simulink model "Assignment1_A1V1"  (R2020a)
settings: Solver=FixedStepAuto  StartTime=0.0  StopTime=10.0  FixedStep=1e-3  RelTol=1e-3  EnableMultiTasking=on
undefined symbols (not defined in the file): D10, D11, D12, D2, D4, D5, D7, D8, D9, PTA0, PTA2, PTB23, PTB9, PTC3, PTC4, PTD0, PTD2, PTD3
libraries: frdmk64flib x12
settings Model: ExtModeTrigDuration=5  Creator=Daniyal  LastModifiedBy=Daniyal
settings OptimizationCC: EnhancedBackFolding=on  PassReuseOutputArgsAs=Individual arguments  ZeroExternalMemoryAtStartup=off  ZeroInternalMemoryAtStartup=off  MaxStackSize=64  OptimizeBlockOrder=speed  DifferentSizesBufferReuse=on  OptimizationCustomize=off  EfficientTunableParamExpr=on
settings DebuggingCC: ParameterTunabilityLossMsg=error
settings HardwareCC: ProdBitPerPointer=32  ProdBitPerSizeT=32  ProdBitPerPtrDiffT=32  ProdLargestAtomicInteger=Long  ProdLargestAtomicFloat=Double  ProdWordSize=32  ProdHWDeviceType=ARM Compatible->ARM Cortex
settings SFSimCC: MATLABDynamicMemAlloc=off
settings RTWCC: SystemTargetFile=ert.tlc  HardwareBoard=NXP FRDM-K64F  TemplateMakefile=ert_default_tmf  Toolchain=GNU Tools for ARM Embedded Processors
settings CodeAppCC: ForceParamTrailComments=on  IgnoreCustomStorageClasses=off  OperatorAnnotations=on  SimulinkDataObjDesc=on  SFDataObjDesc=on  InsertBlockDesc=on

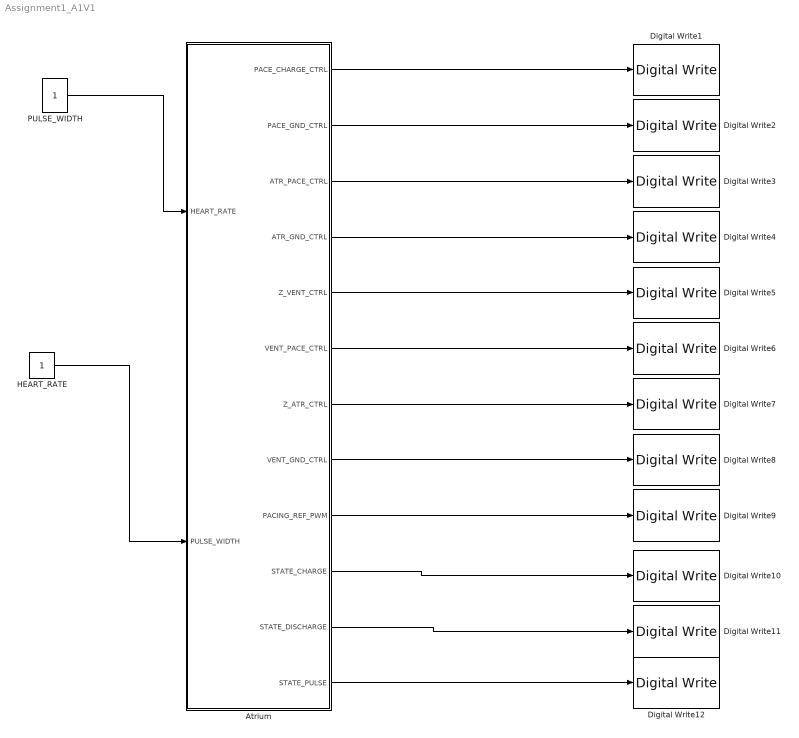
== system Assignment1_A1V1 ==
  Atrium : Stateflow chart  TreatAsAtomicUnit=on
  Digital Write1 : frdmk64flib/Digital Write  Whichpin=PTB9 (D2)
  Digital Write10 : frdmk64flib/Digital Write  Whichpin=RED_LED
  Digital Write11 : frdmk64flib/Digital Write  Whichpin=GREEN_LED
  Digital Write12 : frdmk64flib/Digital Write  Whichpin=BLUE_LED
  Digital Write2 : frdmk64flib/Digital Write  Whichpin=PTD0 (D10)
  Digital Write3 : frdmk64flib/Digital Write  Whichpin=PTA0 (D8)
  Digital Write4 : frdmk64flib/Digital Write  Whichpin=PTD2 (D11)
  Digital Write5 : frdmk64flib/Digital Write  Whichpin=PTC3 (D7)
  Digital Write6 : frdmk64flib/Digital Write  Whichpin=PTC4 (D9)
  Digital Write7 : frdmk64flib/Digital Write  Whichpin=PTB23 (D4)
  Digital Write8 : frdmk64flib/Digital Write  Whichpin=PTD3 (D12)
  Digital Write9 : frdmk64flib/Digital Write  Whichpin=PTA2 (D5)
  HEART_RATE : Constant
  PULSE_WIDTH : Constant
  wires:
  Atrium/4(ATR_GND_CTRL) -> Digital Write4/1
  Atrium/5(Z_VENT_CTRL) -> Digital Write5/1
  Atrium/6(VENT_PACE_CTRL) -> Digital Write6/1
  Atrium/3(ATR_PACE_CTRL) -> Digital Write3/1
  Atrium/8(VENT_GND_CTRL) -> Digital Write8/1
  Atrium/10(STATE_CHARGE) -> Digital Write10/1
  Atrium/11(STATE_DISCHARGE) -> Digital Write11/1
  Atrium/12(STATE_PULSE) -> Digital Write12/1
  Atrium/1(PACE_CHARGE_CTRL) -> Digital Write1/1
  PULSE_WIDTH/1 -> Atrium/1(HEART_RATE)
  Atrium/7(Z_ATR_CTRL) -> Digital Write7/1
  Atrium/9(PACING_REF_PWM) -> Digital Write9/1
  HEART_RATE/1 -> Atrium/2(PULSE_WIDTH)
  Atrium/2(PACE_GND_CTRL) -> Digital Write2/1

== stateflow chart Assignment1_A1V1/Atrium ==
  state CHARGE
    entry:
    during:
    STATE_CHARGE = 1;
    STATE_DISCHARGE = 0;
    STATE_PULSE = 0;
    ATR_PACE_CTRL = 0;
    VENT_PACE_CTRL  = 0;
    PACING_REF_PWM = 2000;
    PACE_CHARGE_CTRL = 1;
    exit:
  state DISCHARGE
    entry:
    during:
    STATE_CHARGE = 0;
    STATE_DISCHARGE = 1;
    STATE_PULSE = 0;
    Z_ATR_CTRL =  0;
    Z_VENT_CTRL =  0;
    ATR_PACE_CTRL =  0;
    ATR_GND_CTRL = 1;
    VENT_GND_CTRL =  0;
    exit:
  state PULSE_ATRIUM
    entry:
    during:
    STATE_CHARGE = 0;
    STATE_DISCHARGE = 0;
    STATE_PULSE = 1;
    PACE_CHARGE_CTRL =  false;
    PACE_GND_CTRL = 1;
    ATR_PACE_CTRL = 1;
    ATR_GND_CTRL =  0;
    Z_ATR_CTRL = 0;
    Z_VENT_CTRL =  0;
    VENT_GND_CTRL =0;
    VENT_PACE_CTRL =  0;
    PACE_GND_CTRL = 1;
    VENT_PACE_CTRL = 0;
    exit:
  (default) -> PULSE_ATRIUM
  CHARGE -> PULSE_ATRIUM : [after(500,msec)]
  PULSE_ATRIUM -> DISCHARGE : [after(500,msec)]
  DISCHARGE -> CHARGE : [after(500,msec)]
  data: HEART_RATE input int16; PULSE_WIDTH input int16; PACE_CHARGE_CTRL output boolean =false; PACE_GND_CTRL output boolean =false; ATR_PACE_CTRL output boolean =false; ATR_GND_CTRL output boolean =false; Z_VENT_CTRL output boolean =false; VENT_PACE_CTRL output boolean =false; Z_ATR_CTRL output boolean =false; VENT_GND_CTRL output boolean =false; PACING_REF_PWM output boolean =false; STATE_CHARGE output boolean; STATE_DISCHARGE output boolean; STATE_PULSE output boolean
